simulink model "simutask"  (R2025b)
settings: Solver=VariableStepAuto  StartTime=0.0  StopTime=10.0  RelTol=1e-3
libraries: simulink x1
settings Model: DataTypeOverride=Double  MinMaxOverflowLogging=ForceOff

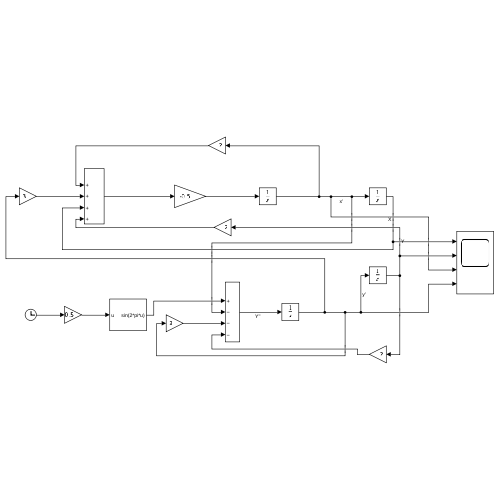
[thumbnail: Simulink's stored preview of the top-level diagram]
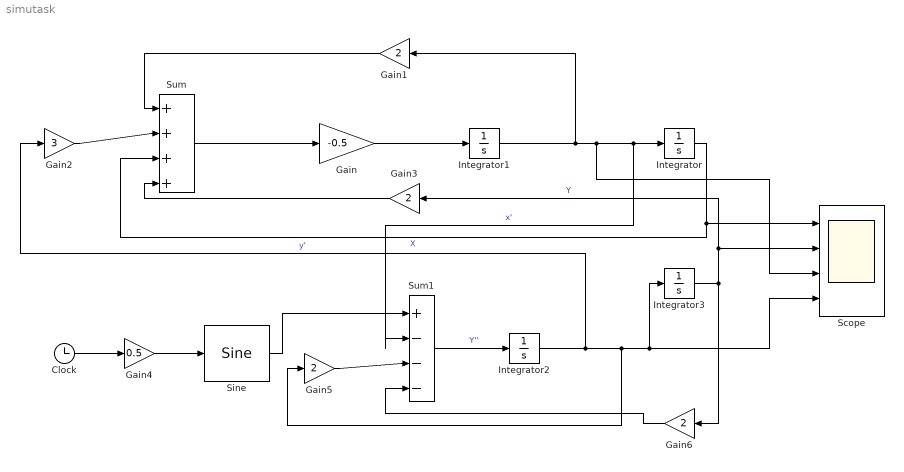
== system simutask ==
  Clock : Clock
  Gain : Gain  Gain=-0.5
  Gain{1,3,5..6} (4 alike) : Gain  Gain=2
  Gain2 : Gain  Gain=3
  Gain4 : Gain  Gain=0.5
  Integrator{,1..3} (4 alike) : Integrator
  Scope : Scope  NumInputPorts=4
  Sine : simulink/Lookup Tables/Sine  Formula=sin(2*pi*u)  NumDataPoints=(2^5)+1  OutputWordLength=16  InternalRulePriority=Speed
  Sum : Sum  Inputs=|++++
  Sum1 : Sum  Inputs=|+---
  wires:
  Integrator1/1 -> Gain1/1, Scope/3, Sum1/2, Integrator/1  "x'"
  Integrator2/1 -> Gain2/1, Gain5/1, Scope/4, Integrator3/1  "y'"
  Gain/1 -> Integrator1/1
  Sum/1 -> Gain/1
  Gain1/1 -> Sum/1
  Gain2/1 -> Sum/2
  Integrator/1 -> Scope/1, Sum/3  "X"
  Integrator3/1 -> Scope/2, Gain3/1, Gain6/1  "Y"
  Gain3/1 -> Sum/4
  Sum1/1 -> Integrator2/1  "Y''"
  Gain4/1 -> Sine/1
  Clock/1 -> Gain4/1
  Sine/1 -> Sum1/1
  Gain5/1 -> Sum1/3
  Gain6/1 -> Sum1/4
